simulink model "StPassCmprtMd_MdXX_CrtStat"  (R2018b)
settings: Solver=FixedStepDiscrete  StartTime=0.0  StopTime=10.0  FixedStep=0.01  RelTol=1e-3
settings Model: Creator=sn2xws  LastModifiedBy=sn2xws
settings DataIOCC: SaveFormat=StructureWithTime
settings OptimizationCC: DefaultParameterBehavior=Inlined  EnhancedBackFolding=on  PassReuseOutputArgsAs=Individual arguments  ZeroExternalMemoryAtStartup=off  ZeroInternalMemoryAtStartup=off  OptimizeBlockOrder=speed  DifferentSizesBufferReuse=on  OptimizationCustomize=off
settings DebuggingCC: ParameterTunabilityLossMsg=error
settings ModelReferenceCC: ModelReferenceNumInstancesAllowed=Single
settings SFSimCC: MATLABDynamicMemAlloc=off
settings RTWCC: SystemTargetFile=autosar.tlc  GenCodeOnly=on  TemplateMakefile=ert_default_tmf  Description=AUTOSAR  GenerateReport=on  IncludeHyperlinkInReport=on  LaunchReport=on  GenerateTraceInfo=on  GenerateTraceReport=on  GenerateTraceReportSl=on  GenerateTraceReportSf=on  GenerateTraceReportEml=on
settings CodeAppCC: ForceParamTrailComments=on  IgnoreCustomStorageClasses=off  OperatorAnnotations=on  SimulinkDataObjDesc=on  SFDataObjDesc=on  InsertBlockDesc=on
settings STFCustomTargetCC: TargetLangStandard=C99 (ISO)  MultiwordLength=256  ParMdlRefBuildCompliant=on  CompOptLevelCompliant=on  IncludeMdlTerminateFcn=off  CombineOutputUpdateFcns=on  SuppressErrorStatus=on  ERTCustomFileBanners=on  SupportNonFinite=off  SupportComplex=off  SupportContinuousTime=off  SupportNonInlinedSFcns=off  RemoveResetFunc=on  MATLABClassNameForMDSCustomization=Simulink.SoftwareTarget.ERTCustomization  AutosarCompliant=on  UseToolchainInfoCompliant=on  LookupTableObjectStructAxisOrder=2,1,3,4,...  LUTObjectStructOrderEvenSpacing=Size,Table,Breakpoints  SystemTargetFile=autosar.tlc
settings ERTTargetCC: TargetLangStandard=C99 (ISO)  ConcurrentExecutionCompliant=off  IncludeMdlTerminateFcn=off  SuppressErrorStatus=on  SupportNonFinite=off  SupportComplex=off  ModelStepFunctionPrototypeControlCompliant=off  CPPClassGenCompliant=off  AutosarCompliant=on  LookupTableObjectStructAxisOrder=2,1,3,4,...  LUTObjectStructOrderEvenSpacing=Size,Table,Breakpoints  InlinedParameterPlacement=NonHierarchical  ERTCustomFileTemplate=example_file_process.tlc

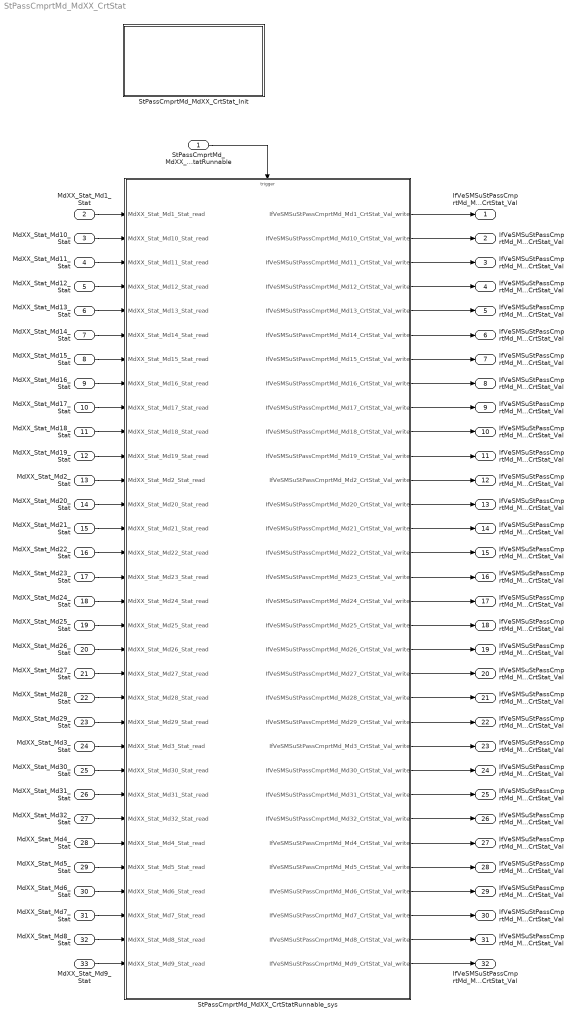
== system StPassCmprtMd_MdXX_CrtStat ==
  StPassCmprtMd_MdXX_CrtStatRunnable : Inport  SampleTime=0.01  OutputFunctionCall=on
  MdXX_Stat_Md1_Stat : Inport  Port=2  OutDataTypeStr=uint8  PortDimensions=1
  MdXX_Stat_Md10_Stat : Inport  Port=3  OutDataTypeStr=uint8  PortDimensions=1
  MdXX_Stat_Md11_Stat : Inport  Port=4  OutDataTypeStr=uint8  PortDimensions=1
  MdXX_Stat_Md12_Stat : Inport  Port=5  OutDataTypeStr=uint8  PortDimensions=1
  MdXX_Stat_Md13_Stat : Inport  Port=6  OutDataTypeStr=uint8  PortDimensions=1
  MdXX_Stat_Md14_Stat : Inport  Port=7  OutDataTypeStr=uint8  PortDimensions=1
  MdXX_Stat_Md15_Stat : Inport  Port=8  OutDataTypeStr=uint8  PortDimensions=1
  MdXX_Stat_Md16_Stat : Inport  Port=9  OutDataTypeStr=uint8  PortDimensions=1
  MdXX_Stat_Md17_Stat : Inport  Port=10  OutDataTypeStr=uint8  PortDimensions=1
  MdXX_Stat_Md18_Stat : Inport  Port=11  OutDataTypeStr=uint8  PortDimensions=1
  MdXX_Stat_Md19_Stat : Inport  Port=12  OutDataTypeStr=uint8  PortDimensions=1
  MdXX_Stat_Md2_Stat : Inport  Port=13  OutDataTypeStr=uint8  PortDimensions=1
  MdXX_Stat_Md20_Stat : Inport  Port=14  OutDataTypeStr=uint8  PortDimensions=1
  MdXX_Stat_Md21_Stat : Inport  Port=15  OutDataTypeStr=uint8  PortDimensions=1
  MdXX_Stat_Md22_Stat : Inport  Port=16  OutDataTypeStr=uint8  PortDimensions=1
  MdXX_Stat_Md23_Stat : Inport  Port=17  OutDataTypeStr=uint8  PortDimensions=1
  MdXX_Stat_Md24_Stat : Inport  Port=18  OutDataTypeStr=uint8  PortDimensions=1
  MdXX_Stat_Md25_Stat : Inport  Port=19  OutDataTypeStr=uint8  PortDimensions=1
  MdXX_Stat_Md26_Stat : Inport  Port=20  OutDataTypeStr=uint8  PortDimensions=1
  MdXX_Stat_Md27_Stat : Inport  Port=21  OutDataTypeStr=uint8  PortDimensions=1
  MdXX_Stat_Md28_Stat : Inport  Port=22  OutDataTypeStr=uint8  PortDimensions=1
  MdXX_Stat_Md29_Stat : Inport  Port=23  OutDataTypeStr=uint8  PortDimensions=1
  MdXX_Stat_Md3_Stat : Inport  Port=24  OutDataTypeStr=uint8  PortDimensions=1
  MdXX_Stat_Md30_Stat : Inport  Port=25  OutDataTypeStr=uint8  PortDimensions=1
  MdXX_Stat_Md31_Stat : Inport  Port=26  OutDataTypeStr=uint8  PortDimensions=1
  MdXX_Stat_Md32_Stat : Inport  Port=27  OutDataTypeStr=uint8  PortDimensions=1
  MdXX_Stat_Md4_Stat : Inport  Port=28  OutDataTypeStr=uint8  PortDimensions=1
  MdXX_Stat_Md5_Stat : Inport  Port=29  OutDataTypeStr=uint8  PortDimensions=1
  MdXX_Stat_Md6_Stat : Inport  Port=30  OutDataTypeStr=uint8  PortDimensions=1
  MdXX_Stat_Md7_Stat : Inport  Port=31  OutDataTypeStr=uint8  PortDimensions=1
  MdXX_Stat_Md8_Stat : Inport  Port=32  OutDataTypeStr=uint8  PortDimensions=1
  MdXX_Stat_Md9_Stat : Inport  Port=33  OutDataTypeStr=uint8  PortDimensions=1
  StPassCmprtMd_MdXX_CrtStatRunnable_sys : Subsystem
  StPassCmprtMd_MdXX_CrtStat_Init : Subsystem
  IfVeSMSuStPassCmprtMd_Md1_CrtStat_Val : Outport  OutDataTypeStr=uint8  PortDimensions=1
  IfVeSMSuStPassCmprtMd_Md10_CrtStat_Val : Outport  Port=2  OutDataTypeStr=uint8  PortDimensions=1
  IfVeSMSuStPassCmprtMd_Md11_CrtStat_Val : Outport  Port=3  OutDataTypeStr=uint8  PortDimensions=1
  IfVeSMSuStPassCmprtMd_Md12_CrtStat_Val : Outport  Port=4  OutDataTypeStr=uint8  PortDimensions=1
  IfVeSMSuStPassCmprtMd_Md13_CrtStat_Val : Outport  Port=5  OutDataTypeStr=uint8  PortDimensions=1
  IfVeSMSuStPassCmprtMd_Md14_CrtStat_Val : Outport  Port=6  OutDataTypeStr=uint8  PortDimensions=1
  IfVeSMSuStPassCmprtMd_Md15_CrtStat_Val : Outport  Port=7  OutDataTypeStr=uint8  PortDimensions=1
  IfVeSMSuStPassCmprtMd_Md16_CrtStat_Val : Outport  Port=8  OutDataTypeStr=uint8  PortDimensions=1
  IfVeSMSuStPassCmprtMd_Md17_CrtStat_Val : Outport  Port=9  OutDataTypeStr=uint8  PortDimensions=1
  IfVeSMSuStPassCmprtMd_Md18_CrtStat_Val : Outport  Port=10  OutDataTypeStr=uint8  PortDimensions=1
  IfVeSMSuStPassCmprtMd_Md19_CrtStat_Val : Outport  Port=11  OutDataTypeStr=uint8  PortDimensions=1
  IfVeSMSuStPassCmprtMd_Md2_CrtStat_Val : Outport  Port=12  OutDataTypeStr=uint8  PortDimensions=1
  IfVeSMSuStPassCmprtMd_Md20_CrtStat_Val : Outport  Port=13  OutDataTypeStr=uint8  PortDimensions=1
  IfVeSMSuStPassCmprtMd_Md21_CrtStat_Val : Outport  Port=14  OutDataTypeStr=uint8  PortDimensions=1
  IfVeSMSuStPassCmprtMd_Md22_CrtStat_Val : Outport  Port=15  OutDataTypeStr=uint8  PortDimensions=1
  IfVeSMSuStPassCmprtMd_Md23_CrtStat_Val : Outport  Port=16  OutDataTypeStr=uint8  PortDimensions=1
  IfVeSMSuStPassCmprtMd_Md24_CrtStat_Val : Outport  Port=17  OutDataTypeStr=uint8  PortDimensions=1
  IfVeSMSuStPassCmprtMd_Md25_CrtStat_Val : Outport  Port=18  OutDataTypeStr=uint8  PortDimensions=1
  IfVeSMSuStPassCmprtMd_Md26_CrtStat_Val : Outport  Port=19  OutDataTypeStr=uint8  PortDimensions=1
  IfVeSMSuStPassCmprtMd_Md27_CrtStat_Val : Outport  Port=20  OutDataTypeStr=uint8  PortDimensions=1
  IfVeSMSuStPassCmprtMd_Md28_CrtStat_Val : Outport  Port=21  OutDataTypeStr=uint8  PortDimensions=1
  IfVeSMSuStPassCmprtMd_Md29_CrtStat_Val : Outport  Port=22  OutDataTypeStr=uint8  PortDimensions=1
  IfVeSMSuStPassCmprtMd_Md3_CrtStat_Val : Outport  Port=23  OutDataTypeStr=uint8  PortDimensions=1
  IfVeSMSuStPassCmprtMd_Md30_CrtStat_Val : Outport  Port=24  OutDataTypeStr=uint8  PortDimensions=1
  IfVeSMSuStPassCmprtMd_Md31_CrtStat_Val : Outport  Port=25  OutDataTypeStr=uint8  PortDimensions=1
  IfVeSMSuStPassCmprtMd_Md32_CrtStat_Val : Outport  Port=26  OutDataTypeStr=uint8  PortDimensions=1
  IfVeSMSuStPassCmprtMd_Md4_CrtStat_Val : Outport  Port=27  OutDataTypeStr=uint8  PortDimensions=1
  IfVeSMSuStPassCmprtMd_Md5_CrtStat_Val : Outport  Port=28  OutDataTypeStr=uint8  PortDimensions=1
  IfVeSMSuStPassCmprtMd_Md6_CrtStat_Val : Outport  Port=29  OutDataTypeStr=uint8  PortDimensions=1
  IfVeSMSuStPassCmprtMd_Md7_CrtStat_Val : Outport  Port=30  OutDataTypeStr=uint8  PortDimensions=1
  IfVeSMSuStPassCmprtMd_Md8_CrtStat_Val : Outport  Port=31  OutDataTypeStr=uint8  PortDimensions=1
  IfVeSMSuStPassCmprtMd_Md9_CrtStat_Val : Outport  Port=32  OutDataTypeStr=uint8  PortDimensions=1
  wires:
  MdXX_Stat_Md1_Stat/1 -> StPassCmprtMd_MdXX_CrtStatRunnable_sys/1(MdXX_Stat_Md1_Stat_read)
  MdXX_Stat_Md10_Stat/1 -> StPassCmprtMd_MdXX_CrtStatRunnable_sys/2(MdXX_Stat_Md10_Stat_read)
  MdXX_Stat_Md11_Stat/1 -> StPassCmprtMd_MdXX_CrtStatRunnable_sys/3(MdXX_Stat_Md11_Stat_read)
  MdXX_Stat_Md12_Stat/1 -> StPassCmprtMd_MdXX_CrtStatRunnable_sys/4(MdXX_Stat_Md12_Stat_read)
  MdXX_Stat_Md13_Stat/1 -> StPassCmprtMd_MdXX_CrtStatRunnable_sys/5(MdXX_Stat_Md13_Stat_read)
  MdXX_Stat_Md14_Stat/1 -> StPassCmprtMd_MdXX_CrtStatRunnable_sys/6(MdXX_Stat_Md14_Stat_read)
  MdXX_Stat_Md15_Stat/1 -> StPassCmprtMd_MdXX_CrtStatRunnable_sys/7(MdXX_Stat_Md15_Stat_read)
  MdXX_Stat_Md16_Stat/1 -> StPassCmprtMd_MdXX_CrtStatRunnable_sys/8(MdXX_Stat_Md16_Stat_read)
  MdXX_Stat_Md17_Stat/1 -> StPassCmprtMd_MdXX_CrtStatRunnable_sys/9(MdXX_Stat_Md17_Stat_read)
  MdXX_Stat_Md18_Stat/1 -> StPassCmprtMd_MdXX_CrtStatRunnable_sys/10(MdXX_Stat_Md18_Stat_read)
  MdXX_Stat_Md19_Stat/1 -> StPassCmprtMd_MdXX_CrtStatRunnable_sys/11(MdXX_Stat_Md19_Stat_read)
  MdXX_Stat_Md2_Stat/1 -> StPassCmprtMd_MdXX_CrtStatRunnable_sys/12(MdXX_Stat_Md2_Stat_read)
  MdXX_Stat_Md20_Stat/1 -> StPassCmprtMd_MdXX_CrtStatRunnable_sys/13(MdXX_Stat_Md20_Stat_read)
  MdXX_Stat_Md21_Stat/1 -> StPassCmprtMd_MdXX_CrtStatRunnable_sys/14(MdXX_Stat_Md21_Stat_read)
  MdXX_Stat_Md22_Stat/1 -> StPassCmprtMd_MdXX_CrtStatRunnable_sys/15(MdXX_Stat_Md22_Stat_read)
  MdXX_Stat_Md23_Stat/1 -> StPassCmprtMd_MdXX_CrtStatRunnable_sys/16(MdXX_Stat_Md23_Stat_read)
  MdXX_Stat_Md24_Stat/1 -> StPassCmprtMd_MdXX_CrtStatRunnable_sys/17(MdXX_Stat_Md24_Stat_read)
  MdXX_Stat_Md25_Stat/1 -> StPassCmprtMd_MdXX_CrtStatRunnable_sys/18(MdXX_Stat_Md25_Stat_read)
  MdXX_Stat_Md26_Stat/1 -> StPassCmprtMd_MdXX_CrtStatRunnable_sys/19(MdXX_Stat_Md26_Stat_read)
  MdXX_Stat_Md27_Stat/1 -> StPassCmprtMd_MdXX_CrtStatRunnable_sys/20(MdXX_Stat_Md27_Stat_read)
  MdXX_Stat_Md28_Stat/1 -> StPassCmprtMd_MdXX_CrtStatRunnable_sys/21(MdXX_Stat_Md28_Stat_read)
  MdXX_Stat_Md29_Stat/1 -> StPassCmprtMd_MdXX_CrtStatRunnable_sys/22(MdXX_Stat_Md29_Stat_read)
  MdXX_Stat_Md3_Stat/1 -> StPassCmprtMd_MdXX_CrtStatRunnable_sys/23(MdXX_Stat_Md3_Stat_read)
  MdXX_Stat_Md30_Stat/1 -> StPassCmprtMd_MdXX_CrtStatRunnable_sys/24(MdXX_Stat_Md30_Stat_read)
  MdXX_Stat_Md31_Stat/1 -> StPassCmprtMd_MdXX_CrtStatRunnable_sys/25(MdXX_Stat_Md31_Stat_read)
  MdXX_Stat_Md32_Stat/1 -> StPassCmprtMd_MdXX_CrtStatRunnable_sys/26(MdXX_Stat_Md32_Stat_read)
  MdXX_Stat_Md4_Stat/1 -> StPassCmprtMd_MdXX_CrtStatRunnable_sys/27(MdXX_Stat_Md4_Stat_read)
  MdXX_Stat_Md5_Stat/1 -> StPassCmprtMd_MdXX_CrtStatRunnable_sys/28(MdXX_Stat_Md5_Stat_read)
  MdXX_Stat_Md6_Stat/1 -> StPassCmprtMd_MdXX_CrtStatRunnable_sys/29(MdXX_Stat_Md6_Stat_read)
  MdXX_Stat_Md7_Stat/1 -> StPassCmprtMd_MdXX_CrtStatRunnable_sys/30(MdXX_Stat_Md7_Stat_read)
  MdXX_Stat_Md8_Stat/1 -> StPassCmprtMd_MdXX_CrtStatRunnable_sys/31(MdXX_Stat_Md8_Stat_read)
  MdXX_Stat_Md9_Stat/1 -> StPassCmprtMd_MdXX_CrtStatRunnable_sys/32(MdXX_Stat_Md9_Stat_read)
  StPassCmprtMd_MdXX_CrtStatRunnable_sys/1(IfVeSMSuStPassCmprtMd_Md1_CrtStat_Val_write) -> IfVeSMSuStPassCmprtMd_Md1_CrtStat_Val/1
  StPassCmprtMd_MdXX_CrtStatRunnable_sys/2(IfVeSMSuStPassCmprtMd_Md10_CrtStat_Val_write) -> IfVeSMSuStPassCmprtMd_Md10_CrtStat_Val/1
  StPassCmprtMd_MdXX_CrtStatRunnable_sys/3(IfVeSMSuStPassCmprtMd_Md11_CrtStat_Val_write) -> IfVeSMSuStPassCmprtMd_Md11_CrtStat_Val/1
  StPassCmprtMd_MdXX_CrtStatRunnable_sys/4(IfVeSMSuStPassCmprtMd_Md12_CrtStat_Val_write) -> IfVeSMSuStPassCmprtMd_Md12_CrtStat_Val/1
  StPassCmprtMd_MdXX_CrtStatRunnable_sys/5(IfVeSMSuStPassCmprtMd_Md13_CrtStat_Val_write) -> IfVeSMSuStPassCmprtMd_Md13_CrtStat_Val/1
  StPassCmprtMd_MdXX_CrtStatRunnable_sys/6(IfVeSMSuStPassCmprtMd_Md14_CrtStat_Val_write) -> IfVeSMSuStPassCmprtMd_Md14_CrtStat_Val/1
  StPassCmprtMd_MdXX_CrtStatRunnable_sys/7(IfVeSMSuStPassCmprtMd_Md15_CrtStat_Val_write) -> IfVeSMSuStPassCmprtMd_Md15_CrtStat_Val/1
  StPassCmprtMd_MdXX_CrtStatRunnable_sys/8(IfVeSMSuStPassCmprtMd_Md16_CrtStat_Val_write) -> IfVeSMSuStPassCmprtMd_Md16_CrtStat_Val/1
  StPassCmprtMd_MdXX_CrtStatRunnable_sys/9(IfVeSMSuStPassCmprtMd_Md17_CrtStat_Val_write) -> IfVeSMSuStPassCmprtMd_Md17_CrtStat_Val/1
  StPassCmprtMd_MdXX_CrtStatRunnable_sys/10(IfVeSMSuStPassCmprtMd_Md18_CrtStat_Val_write) -> IfVeSMSuStPassCmprtMd_Md18_CrtStat_Val/1
  StPassCmprtMd_MdXX_CrtStatRunnable_sys/11(IfVeSMSuStPassCmprtMd_Md19_CrtStat_Val_write) -> IfVeSMSuStPassCmprtMd_Md19_CrtStat_Val/1
  StPassCmprtMd_MdXX_CrtStatRunnable_sys/12(IfVeSMSuStPassCmprtMd_Md2_CrtStat_Val_write) -> IfVeSMSuStPassCmprtMd_Md2_CrtStat_Val/1
  StPassCmprtMd_MdXX_CrtStatRunnable_sys/13(IfVeSMSuStPassCmprtMd_Md20_CrtStat_Val_write) -> IfVeSMSuStPassCmprtMd_Md20_CrtStat_Val/1
  StPassCmprtMd_MdXX_CrtStatRunnable_sys/14(IfVeSMSuStPassCmprtMd_Md21_CrtStat_Val_write) -> IfVeSMSuStPassCmprtMd_Md21_CrtStat_Val/1
  StPassCmprtMd_MdXX_CrtStatRunnable_sys/15(IfVeSMSuStPassCmprtMd_Md22_CrtStat_Val_write) -> IfVeSMSuStPassCmprtMd_Md22_CrtStat_Val/1
  StPassCmprtMd_MdXX_CrtStatRunnable_sys/16(IfVeSMSuStPassCmprtMd_Md23_CrtStat_Val_write) -> IfVeSMSuStPassCmprtMd_Md23_CrtStat_Val/1
  StPassCmprtMd_MdXX_CrtStatRunnable_sys/17(IfVeSMSuStPassCmprtMd_Md24_CrtStat_Val_write) -> IfVeSMSuStPassCmprtMd_Md24_CrtStat_Val/1
  StPassCmprtMd_MdXX_CrtStatRunnable_sys/18(IfVeSMSuStPassCmprtMd_Md25_CrtStat_Val_write) -> IfVeSMSuStPassCmprtMd_Md25_CrtStat_Val/1
  StPassCmprtMd_MdXX_CrtStatRunnable_sys/19(IfVeSMSuStPassCmprtMd_Md26_CrtStat_Val_write) -> IfVeSMSuStPassCmprtMd_Md26_CrtStat_Val/1
  StPassCmprtMd_MdXX_CrtStatRunnable_sys/20(IfVeSMSuStPassCmprtMd_Md27_CrtStat_Val_write) -> IfVeSMSuStPassCmprtMd_Md27_CrtStat_Val/1
  StPassCmprtMd_MdXX_CrtStatRunnable_sys/21(IfVeSMSuStPassCmprtMd_Md28_CrtStat_Val_write) -> IfVeSMSuStPassCmprtMd_Md28_CrtStat_Val/1
  StPassCmprtMd_MdXX_CrtStatRunnable_sys/22(IfVeSMSuStPassCmprtMd_Md29_CrtStat_Val_write) -> IfVeSMSuStPassCmprtMd_Md29_CrtStat_Val/1
  StPassCmprtMd_MdXX_CrtStatRunnable_sys/23(IfVeSMSuStPassCmprtMd_Md3_CrtStat_Val_write) -> IfVeSMSuStPassCmprtMd_Md3_CrtStat_Val/1
  StPassCmprtMd_MdXX_CrtStatRunnable_sys/24(IfVeSMSuStPassCmprtMd_Md30_CrtStat_Val_write) -> IfVeSMSuStPassCmprtMd_Md30_CrtStat_Val/1
  StPassCmprtMd_MdXX_CrtStatRunnable_sys/25(IfVeSMSuStPassCmprtMd_Md31_CrtStat_Val_write) -> IfVeSMSuStPassCmprtMd_Md31_CrtStat_Val/1
  StPassCmprtMd_MdXX_CrtStatRunnable_sys/26(IfVeSMSuStPassCmprtMd_Md32_CrtStat_Val_write) -> IfVeSMSuStPassCmprtMd_Md32_CrtStat_Val/1
  StPassCmprtMd_MdXX_CrtStatRunnable_sys/27(IfVeSMSuStPassCmprtMd_Md4_CrtStat_Val_write) -> IfVeSMSuStPassCmprtMd_Md4_CrtStat_Val/1
  StPassCmprtMd_MdXX_CrtStatRunnable_sys/28(IfVeSMSuStPassCmprtMd_Md5_CrtStat_Val_write) -> IfVeSMSuStPassCmprtMd_Md5_CrtStat_Val/1
  StPassCmprtMd_MdXX_CrtStatRunnable_sys/29(IfVeSMSuStPassCmprtMd_Md6_CrtStat_Val_write) -> IfVeSMSuStPassCmprtMd_Md6_CrtStat_Val/1
  StPassCmprtMd_MdXX_CrtStatRunnable_sys/30(IfVeSMSuStPassCmprtMd_Md7_CrtStat_Val_write) -> IfVeSMSuStPassCmprtMd_Md7_CrtStat_Val/1
  StPassCmprtMd_MdXX_CrtStatRunnable_sys/31(IfVeSMSuStPassCmprtMd_Md8_CrtStat_Val_write) -> IfVeSMSuStPassCmprtMd_Md8_CrtStat_Val/1
  StPassCmprtMd_MdXX_CrtStatRunnable_sys/32(IfVeSMSuStPassCmprtMd_Md9_CrtStat_Val_write) -> IfVeSMSuStPassCmprtMd_Md9_CrtStat_Val/1
  StPassCmprtMd_MdXX_CrtStatRunnable/1 -> StPassCmprtMd_MdXX_CrtStatRunnable_sys/Trigger

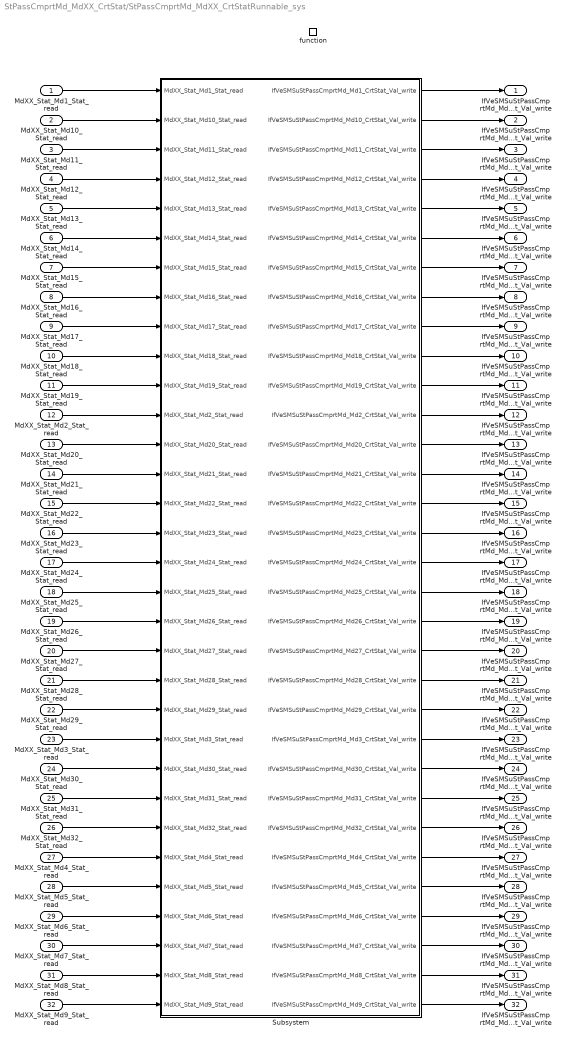
== system StPassCmprtMd_MdXX_CrtStat/StPassCmprtMd_MdXX_CrtStatRunnable_sys ==
  MdXX_Stat_Md1_Stat_read : Inport
  MdXX_Stat_Md10_Stat_read : Inport  Port=2
  MdXX_Stat_Md11_Stat_read : Inport  Port=3
  MdXX_Stat_Md12_Stat_read : Inport  Port=4
  MdXX_Stat_Md13_Stat_read : Inport  Port=5
  MdXX_Stat_Md14_Stat_read : Inport  Port=6
  MdXX_Stat_Md15_Stat_read : Inport  Port=7
  MdXX_Stat_Md16_Stat_read : Inport  Port=8
  MdXX_Stat_Md17_Stat_read : Inport  Port=9
  MdXX_Stat_Md18_Stat_read : Inport  Port=10
  MdXX_Stat_Md19_Stat_read : Inport  Port=11
  MdXX_Stat_Md2_Stat_read : Inport  Port=12
  MdXX_Stat_Md20_Stat_read : Inport  Port=13
  MdXX_Stat_Md21_Stat_read : Inport  Port=14
  MdXX_Stat_Md22_Stat_read : Inport  Port=15
  MdXX_Stat_Md23_Stat_read : Inport  Port=16
  MdXX_Stat_Md24_Stat_read : Inport  Port=17
  MdXX_Stat_Md25_Stat_read : Inport  Port=18
  MdXX_Stat_Md26_Stat_read : Inport  Port=19
  MdXX_Stat_Md27_Stat_read : Inport  Port=20
  MdXX_Stat_Md28_Stat_read : Inport  Port=21
  MdXX_Stat_Md29_Stat_read : Inport  Port=22
  MdXX_Stat_Md3_Stat_read : Inport  Port=23
  MdXX_Stat_Md30_Stat_read : Inport  Port=24
  MdXX_Stat_Md31_Stat_read : Inport  Port=25
  MdXX_Stat_Md32_Stat_read : Inport  Port=26
  MdXX_Stat_Md4_Stat_read : Inport  Port=27
  MdXX_Stat_Md5_Stat_read : Inport  Port=28
  MdXX_Stat_Md6_Stat_read : Inport  Port=29
  MdXX_Stat_Md7_Stat_read : Inport  Port=30
  MdXX_Stat_Md8_Stat_read : Inport  Port=31
  MdXX_Stat_Md9_Stat_read : Inport  Port=32
  function : TriggerPort  TriggerType=function-call  VariantControl=(inherit)  SampleTimeType=periodic  SampleTime=-1
  Subsystem : Subsystem
  IfVeSMSuStPassCmprtMd_Md1_CrtStat_Val_write : Outport
      settings: EnsureOutportIsVirtual=on
  IfVeSMSuStPassCmprtMd_Md10_CrtStat_Val_write : Outport  Port=2
      settings: EnsureOutportIsVirtual=on
  IfVeSMSuStPassCmprtMd_Md11_CrtStat_Val_write : Outport  Port=3
      settings: EnsureOutportIsVirtual=on
  IfVeSMSuStPassCmprtMd_Md12_CrtStat_Val_write : Outport  Port=4
      settings: EnsureOutportIsVirtual=on
  IfVeSMSuStPassCmprtMd_Md13_CrtStat_Val_write : Outport  Port=5
      settings: EnsureOutportIsVirtual=on
  IfVeSMSuStPassCmprtMd_Md14_CrtStat_Val_write : Outport  Port=6
      settings: EnsureOutportIsVirtual=on
  IfVeSMSuStPassCmprtMd_Md15_CrtStat_Val_write : Outport  Port=7
      settings: EnsureOutportIsVirtual=on
  IfVeSMSuStPassCmprtMd_Md16_CrtStat_Val_write : Outport  Port=8
      settings: EnsureOutportIsVirtual=on
  IfVeSMSuStPassCmprtMd_Md17_CrtStat_Val_write : Outport  Port=9
      settings: EnsureOutportIsVirtual=on
  IfVeSMSuStPassCmprtMd_Md18_CrtStat_Val_write : Outport  Port=10
      settings: EnsureOutportIsVirtual=on
  IfVeSMSuStPassCmprtMd_Md19_CrtStat_Val_write : Outport  Port=11
      settings: EnsureOutportIsVirtual=on
  IfVeSMSuStPassCmprtMd_Md2_CrtStat_Val_write : Outport  Port=12
      settings: EnsureOutportIsVirtual=on
  IfVeSMSuStPassCmprtMd_Md20_CrtStat_Val_write : Outport  Port=13
      settings: EnsureOutportIsVirtual=on
  IfVeSMSuStPassCmprtMd_Md21_CrtStat_Val_write : Outport  Port=14
      settings: EnsureOutportIsVirtual=on
  IfVeSMSuStPassCmprtMd_Md22_CrtStat_Val_write : Outport  Port=15
      settings: EnsureOutportIsVirtual=on
  IfVeSMSuStPassCmprtMd_Md23_CrtStat_Val_write : Outport  Port=16
      settings: EnsureOutportIsVirtual=on
  IfVeSMSuStPassCmprtMd_Md24_CrtStat_Val_write : Outport  Port=17
      settings: EnsureOutportIsVirtual=on
  IfVeSMSuStPassCmprtMd_Md25_CrtStat_Val_write : Outport  Port=18
      settings: EnsureOutportIsVirtual=on
  IfVeSMSuStPassCmprtMd_Md26_CrtStat_Val_write : Outport  Port=19
      settings: EnsureOutportIsVirtual=on
  IfVeSMSuStPassCmprtMd_Md27_CrtStat_Val_write : Outport  Port=20
      settings: EnsureOutportIsVirtual=on
  IfVeSMSuStPassCmprtMd_Md28_CrtStat_Val_write : Outport  Port=21
      settings: EnsureOutportIsVirtual=on
  IfVeSMSuStPassCmprtMd_Md29_CrtStat_Val_write : Outport  Port=22
      settings: EnsureOutportIsVirtual=on
  IfVeSMSuStPassCmprtMd_Md3_CrtStat_Val_write : Outport  Port=23
      settings: EnsureOutportIsVirtual=on
  IfVeSMSuStPassCmprtMd_Md30_CrtStat_Val_write : Outport  Port=24
      settings: EnsureOutportIsVirtual=on
  IfVeSMSuStPassCmprtMd_Md31_CrtStat_Val_write : Outport  Port=25
      settings: EnsureOutportIsVirtual=on
  IfVeSMSuStPassCmprtMd_Md32_CrtStat_Val_write : Outport  Port=26
      settings: EnsureOutportIsVirtual=on
  IfVeSMSuStPassCmprtMd_Md4_CrtStat_Val_write : Outport  Port=27
      settings: EnsureOutportIsVirtual=on
  IfVeSMSuStPassCmprtMd_Md5_CrtStat_Val_write : Outport  Port=28
      settings: EnsureOutportIsVirtual=on
  IfVeSMSuStPassCmprtMd_Md6_CrtStat_Val_write : Outport  Port=29
      settings: EnsureOutportIsVirtual=on
  IfVeSMSuStPassCmprtMd_Md7_CrtStat_Val_write : Outport  Port=30
      settings: EnsureOutportIsVirtual=on
  IfVeSMSuStPassCmprtMd_Md8_CrtStat_Val_write : Outport  Port=31
      settings: EnsureOutportIsVirtual=on
  IfVeSMSuStPassCmprtMd_Md9_CrtStat_Val_write : Outport  Port=32
      settings: EnsureOutportIsVirtual=on
  wires:
  MdXX_Stat_Md1_Stat_read/1 -> Subsystem/1(MdXX_Stat_Md1_Stat_read)
  MdXX_Stat_Md10_Stat_read/1 -> Subsystem/2(MdXX_Stat_Md10_Stat_read)
  MdXX_Stat_Md11_Stat_read/1 -> Subsystem/3(MdXX_Stat_Md11_Stat_read)
  MdXX_Stat_Md12_Stat_read/1 -> Subsystem/4(MdXX_Stat_Md12_Stat_read)
  MdXX_Stat_Md13_Stat_read/1 -> Subsystem/5(MdXX_Stat_Md13_Stat_read)
  MdXX_Stat_Md14_Stat_read/1 -> Subsystem/6(MdXX_Stat_Md14_Stat_read)
  MdXX_Stat_Md15_Stat_read/1 -> Subsystem/7(MdXX_Stat_Md15_Stat_read)
  MdXX_Stat_Md16_Stat_read/1 -> Subsystem/8(MdXX_Stat_Md16_Stat_read)
  MdXX_Stat_Md17_Stat_read/1 -> Subsystem/9(MdXX_Stat_Md17_Stat_read)
  MdXX_Stat_Md18_Stat_read/1 -> Subsystem/10(MdXX_Stat_Md18_Stat_read)
  MdXX_Stat_Md19_Stat_read/1 -> Subsystem/11(MdXX_Stat_Md19_Stat_read)
  MdXX_Stat_Md2_Stat_read/1 -> Subsystem/12(MdXX_Stat_Md2_Stat_read)
  MdXX_Stat_Md20_Stat_read/1 -> Subsystem/13(MdXX_Stat_Md20_Stat_read)
  MdXX_Stat_Md21_Stat_read/1 -> Subsystem/14(MdXX_Stat_Md21_Stat_read)
  MdXX_Stat_Md22_Stat_read/1 -> Subsystem/15(MdXX_Stat_Md22_Stat_read)
  MdXX_Stat_Md23_Stat_read/1 -> Subsystem/16(MdXX_Stat_Md23_Stat_read)
  MdXX_Stat_Md24_Stat_read/1 -> Subsystem/17(MdXX_Stat_Md24_Stat_read)
  MdXX_Stat_Md25_Stat_read/1 -> Subsystem/18(MdXX_Stat_Md25_Stat_read)
  MdXX_Stat_Md26_Stat_read/1 -> Subsystem/19(MdXX_Stat_Md26_Stat_read)
  MdXX_Stat_Md27_Stat_read/1 -> Subsystem/20(MdXX_Stat_Md27_Stat_read)
  MdXX_Stat_Md28_Stat_read/1 -> Subsystem/21(MdXX_Stat_Md28_Stat_read)
  MdXX_Stat_Md29_Stat_read/1 -> Subsystem/22(MdXX_Stat_Md29_Stat_read)
  MdXX_Stat_Md3_Stat_read/1 -> Subsystem/23(MdXX_Stat_Md3_Stat_read)
  MdXX_Stat_Md30_Stat_read/1 -> Subsystem/24(MdXX_Stat_Md30_Stat_read)
  MdXX_Stat_Md31_Stat_read/1 -> Subsystem/25(MdXX_Stat_Md31_Stat_read)
  MdXX_Stat_Md32_Stat_read/1 -> Subsystem/26(MdXX_Stat_Md32_Stat_read)
  MdXX_Stat_Md4_Stat_read/1 -> Subsystem/27(MdXX_Stat_Md4_Stat_read)
  MdXX_Stat_Md5_Stat_read/1 -> Subsystem/28(MdXX_Stat_Md5_Stat_read)
  MdXX_Stat_Md6_Stat_read/1 -> Subsystem/29(MdXX_Stat_Md6_Stat_read)
  MdXX_Stat_Md7_Stat_read/1 -> Subsystem/30(MdXX_Stat_Md7_Stat_read)
  MdXX_Stat_Md8_Stat_read/1 -> Subsystem/31(MdXX_Stat_Md8_Stat_read)
  MdXX_Stat_Md9_Stat_read/1 -> Subsystem/32(MdXX_Stat_Md9_Stat_read)
  Subsystem/1(IfVeSMSuStPassCmprtMd_Md1_CrtStat_Val_write) -> IfVeSMSuStPassCmprtMd_Md1_CrtStat_Val_write/1
  Subsystem/2(IfVeSMSuStPassCmprtMd_Md10_CrtStat_Val_write) -> IfVeSMSuStPassCmprtMd_Md10_CrtStat_Val_write/1
  Subsystem/3(IfVeSMSuStPassCmprtMd_Md11_CrtStat_Val_write) -> IfVeSMSuStPassCmprtMd_Md11_CrtStat_Val_write/1
  Subsystem/4(IfVeSMSuStPassCmprtMd_Md12_CrtStat_Val_write) -> IfVeSMSuStPassCmprtMd_Md12_CrtStat_Val_write/1
  Subsystem/5(IfVeSMSuStPassCmprtMd_Md13_CrtStat_Val_write) -> IfVeSMSuStPassCmprtMd_Md13_CrtStat_Val_write/1
  Subsystem/6(IfVeSMSuStPassCmprtMd_Md14_CrtStat_Val_write) -> IfVeSMSuStPassCmprtMd_Md14_CrtStat_Val_write/1
  Subsystem/7(IfVeSMSuStPassCmprtMd_Md15_CrtStat_Val_write) -> IfVeSMSuStPassCmprtMd_Md15_CrtStat_Val_write/1
  Subsystem/8(IfVeSMSuStPassCmprtMd_Md16_CrtStat_Val_write) -> IfVeSMSuStPassCmprtMd_Md16_CrtStat_Val_write/1
  Subsystem/9(IfVeSMSuStPassCmprtMd_Md17_CrtStat_Val_write) -> IfVeSMSuStPassCmprtMd_Md17_CrtStat_Val_write/1
  Subsystem/10(IfVeSMSuStPassCmprtMd_Md18_CrtStat_Val_write) -> IfVeSMSuStPassCmprtMd_Md18_CrtStat_Val_write/1
  Subsystem/11(IfVeSMSuStPassCmprtMd_Md19_CrtStat_Val_write) -> IfVeSMSuStPassCmprtMd_Md19_CrtStat_Val_write/1
  Subsystem/12(IfVeSMSuStPassCmprtMd_Md2_CrtStat_Val_write) -> IfVeSMSuStPassCmprtMd_Md2_CrtStat_Val_write/1
  Subsystem/13(IfVeSMSuStPassCmprtMd_Md20_CrtStat_Val_write) -> IfVeSMSuStPassCmprtMd_Md20_CrtStat_Val_write/1
  Subsystem/14(IfVeSMSuStPassCmprtMd_Md21_CrtStat_Val_write) -> IfVeSMSuStPassCmprtMd_Md21_CrtStat_Val_write/1
  Subsystem/15(IfVeSMSuStPassCmprtMd_Md22_CrtStat_Val_write) -> IfVeSMSuStPassCmprtMd_Md22_CrtStat_Val_write/1
  Subsystem/16(IfVeSMSuStPassCmprtMd_Md23_CrtStat_Val_write) -> IfVeSMSuStPassCmprtMd_Md23_CrtStat_Val_write/1
  Subsystem/17(IfVeSMSuStPassCmprtMd_Md24_CrtStat_Val_write) -> IfVeSMSuStPassCmprtMd_Md24_CrtStat_Val_write/1
  Subsystem/18(IfVeSMSuStPassCmprtMd_Md25_CrtStat_Val_write) -> IfVeSMSuStPassCmprtMd_Md25_CrtStat_Val_write/1
  Subsystem/19(IfVeSMSuStPassCmprtMd_Md26_CrtStat_Val_write) -> IfVeSMSuStPassCmprtMd_Md26_CrtStat_Val_write/1
  Subsystem/20(IfVeSMSuStPassCmprtMd_Md27_CrtStat_Val_write) -> IfVeSMSuStPassCmprtMd_Md27_CrtStat_Val_write/1
  Subsystem/21(IfVeSMSuStPassCmprtMd_Md28_CrtStat_Val_write) -> IfVeSMSuStPassCmprtMd_Md28_CrtStat_Val_write/1
  Subsystem/22(IfVeSMSuStPassCmprtMd_Md29_CrtStat_Val_write) -> IfVeSMSuStPassCmprtMd_Md29_CrtStat_Val_write/1
  Subsystem/23(IfVeSMSuStPassCmprtMd_Md3_CrtStat_Val_write) -> IfVeSMSuStPassCmprtMd_Md3_CrtStat_Val_write/1
  Subsystem/24(IfVeSMSuStPassCmprtMd_Md30_CrtStat_Val_write) -> IfVeSMSuStPassCmprtMd_Md30_CrtStat_Val_write/1
  Subsystem/25(IfVeSMSuStPassCmprtMd_Md31_CrtStat_Val_write) -> IfVeSMSuStPassCmprtMd_Md31_CrtStat_Val_write/1
  Subsystem/26(IfVeSMSuStPassCmprtMd_Md32_CrtStat_Val_write) -> IfVeSMSuStPassCmprtMd_Md32_CrtStat_Val_write/1
  Subsystem/27(IfVeSMSuStPassCmprtMd_Md4_CrtStat_Val_write) -> IfVeSMSuStPassCmprtMd_Md4_CrtStat_Val_write/1
  Subsystem/28(IfVeSMSuStPassCmprtMd_Md5_CrtStat_Val_write) -> IfVeSMSuStPassCmprtMd_Md5_CrtStat_Val_write/1
  Subsystem/29(IfVeSMSuStPassCmprtMd_Md6_CrtStat_Val_write) -> IfVeSMSuStPassCmprtMd_Md6_CrtStat_Val_write/1
  Subsystem/30(IfVeSMSuStPassCmprtMd_Md7_CrtStat_Val_write) -> IfVeSMSuStPassCmprtMd_Md7_CrtStat_Val_write/1
  Subsystem/31(IfVeSMSuStPassCmprtMd_Md8_CrtStat_Val_write) -> IfVeSMSuStPassCmprtMd_Md8_CrtStat_Val_write/1
  Subsystem/32(IfVeSMSuStPassCmprtMd_Md9_CrtStat_Val_write) -> IfVeSMSuStPassCmprtMd_Md9_CrtStat_Val_write/1

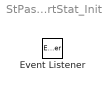
== system StPassCmprtMd_MdXX_CrtStat/StPassCmprtMd_MdXX_CrtStat_Init ==
  Event Listener : EventListener  EventName=reset

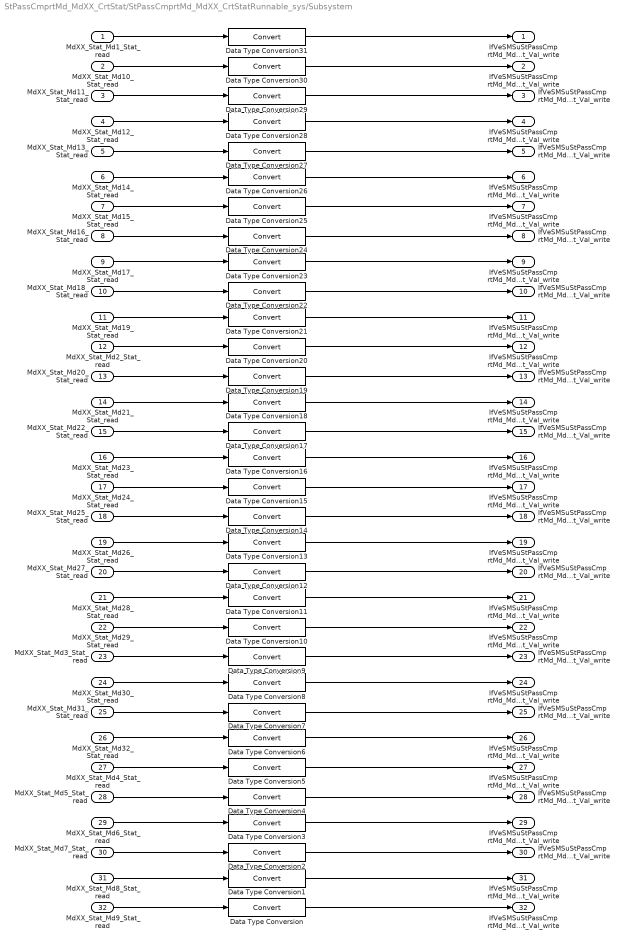
== system StPassCmprtMd_MdXX_CrtStat/StPassCmprtMd_MdXX_CrtStatRunnable_sys/Subsystem ==
  MdXX_Stat_Md1_Stat_read : Inport
  MdXX_Stat_Md10_Stat_read : Inport  Port=2
  MdXX_Stat_Md11_Stat_read : Inport  Port=3
  MdXX_Stat_Md12_Stat_read : Inport  Port=4
  MdXX_Stat_Md13_Stat_read : Inport  Port=5
  MdXX_Stat_Md14_Stat_read : Inport  Port=6
  MdXX_Stat_Md15_Stat_read : Inport  Port=7
  MdXX_Stat_Md16_Stat_read : Inport  Port=8
  MdXX_Stat_Md17_Stat_read : Inport  Port=9
  MdXX_Stat_Md18_Stat_read : Inport  Port=10
  MdXX_Stat_Md19_Stat_read : Inport  Port=11
  MdXX_Stat_Md2_Stat_read : Inport  Port=12
  MdXX_Stat_Md20_Stat_read : Inport  Port=13
  MdXX_Stat_Md21_Stat_read : Inport  Port=14
  MdXX_Stat_Md22_Stat_read : Inport  Port=15
  MdXX_Stat_Md23_Stat_read : Inport  Port=16
  MdXX_Stat_Md24_Stat_read : Inport  Port=17
  MdXX_Stat_Md25_Stat_read : Inport  Port=18
  MdXX_Stat_Md26_Stat_read : Inport  Port=19
  MdXX_Stat_Md27_Stat_read : Inport  Port=20
  MdXX_Stat_Md28_Stat_read : Inport  Port=21
  MdXX_Stat_Md29_Stat_read : Inport  Port=22
  MdXX_Stat_Md3_Stat_read : Inport  Port=23
  MdXX_Stat_Md30_Stat_read : Inport  Port=24
  MdXX_Stat_Md31_Stat_read : Inport  Port=25
  MdXX_Stat_Md32_Stat_read : Inport  Port=26
  MdXX_Stat_Md4_Stat_read : Inport  Port=27
  MdXX_Stat_Md5_Stat_read : Inport  Port=28
  MdXX_Stat_Md6_Stat_read : Inport  Port=29
  MdXX_Stat_Md7_Stat_read : Inport  Port=30
  MdXX_Stat_Md8_Stat_read : Inport  Port=31
  MdXX_Stat_Md9_Stat_read : Inport  Port=32
  Data Type Conversion{,1..31} (32 alike) : DataTypeConversion
  IfVeSMSuStPassCmprtMd_Md1_CrtStat_Val_write : Outport
      settings: EnsureOutportIsVirtual=on
  IfVeSMSuStPassCmprtMd_Md10_CrtStat_Val_write : Outport  Port=2
      settings: EnsureOutportIsVirtual=on
  IfVeSMSuStPassCmprtMd_Md11_CrtStat_Val_write : Outport  Port=3
      settings: EnsureOutportIsVirtual=on
  IfVeSMSuStPassCmprtMd_Md12_CrtStat_Val_write : Outport  Port=4
      settings: EnsureOutportIsVirtual=on
  IfVeSMSuStPassCmprtMd_Md13_CrtStat_Val_write : Outport  Port=5
      settings: EnsureOutportIsVirtual=on
  IfVeSMSuStPassCmprtMd_Md14_CrtStat_Val_write : Outport  Port=6
      settings: EnsureOutportIsVirtual=on
  IfVeSMSuStPassCmprtMd_Md15_CrtStat_Val_write : Outport  Port=7
      settings: EnsureOutportIsVirtual=on
  IfVeSMSuStPassCmprtMd_Md16_CrtStat_Val_write : Outport  Port=8
      settings: EnsureOutportIsVirtual=on
  IfVeSMSuStPassCmprtMd_Md17_CrtStat_Val_write : Outport  Port=9
      settings: EnsureOutportIsVirtual=on
  IfVeSMSuStPassCmprtMd_Md18_CrtStat_Val_write : Outport  Port=10
      settings: EnsureOutportIsVirtual=on
  IfVeSMSuStPassCmprtMd_Md19_CrtStat_Val_write : Outport  Port=11
      settings: EnsureOutportIsVirtual=on
  IfVeSMSuStPassCmprtMd_Md2_CrtStat_Val_write : Outport  Port=12
      settings: EnsureOutportIsVirtual=on
  IfVeSMSuStPassCmprtMd_Md20_CrtStat_Val_write : Outport  Port=13
      settings: EnsureOutportIsVirtual=on
  IfVeSMSuStPassCmprtMd_Md21_CrtStat_Val_write : Outport  Port=14
      settings: EnsureOutportIsVirtual=on
  IfVeSMSuStPassCmprtMd_Md22_CrtStat_Val_write : Outport  Port=15
      settings: EnsureOutportIsVirtual=on
  IfVeSMSuStPassCmprtMd_Md23_CrtStat_Val_write : Outport  Port=16
      settings: EnsureOutportIsVirtual=on
  IfVeSMSuStPassCmprtMd_Md24_CrtStat_Val_write : Outport  Port=17
      settings: EnsureOutportIsVirtual=on
  IfVeSMSuStPassCmprtMd_Md25_CrtStat_Val_write : Outport  Port=18
      settings: EnsureOutportIsVirtual=on
  IfVeSMSuStPassCmprtMd_Md26_CrtStat_Val_write : Outport  Port=19
      settings: EnsureOutportIsVirtual=on
  IfVeSMSuStPassCmprtMd_Md27_CrtStat_Val_write : Outport  Port=20
      settings: EnsureOutportIsVirtual=on
  IfVeSMSuStPassCmprtMd_Md28_CrtStat_Val_write : Outport  Port=21
      settings: EnsureOutportIsVirtual=on
  IfVeSMSuStPassCmprtMd_Md29_CrtStat_Val_write : Outport  Port=22
      settings: EnsureOutportIsVirtual=on
  IfVeSMSuStPassCmprtMd_Md3_CrtStat_Val_write : Outport  Port=23
      settings: EnsureOutportIsVirtual=on
  IfVeSMSuStPassCmprtMd_Md30_CrtStat_Val_write : Outport  Port=24
      settings: EnsureOutportIsVirtual=on
  IfVeSMSuStPassCmprtMd_Md31_CrtStat_Val_write : Outport  Port=25
      settings: EnsureOutportIsVirtual=on
  IfVeSMSuStPassCmprtMd_Md32_CrtStat_Val_write : Outport  Port=26
      settings: EnsureOutportIsVirtual=on
  IfVeSMSuStPassCmprtMd_Md4_CrtStat_Val_write : Outport  Port=27
      settings: EnsureOutportIsVirtual=on
  IfVeSMSuStPassCmprtMd_Md5_CrtStat_Val_write : Outport  Port=28
      settings: EnsureOutportIsVirtual=on
  IfVeSMSuStPassCmprtMd_Md6_CrtStat_Val_write : Outport  Port=29
      settings: EnsureOutportIsVirtual=on
  IfVeSMSuStPassCmprtMd_Md7_CrtStat_Val_write : Outport  Port=30
      settings: EnsureOutportIsVirtual=on
  IfVeSMSuStPassCmprtMd_Md8_CrtStat_Val_write : Outport  Port=31
      settings: EnsureOutportIsVirtual=on
  IfVeSMSuStPassCmprtMd_Md9_CrtStat_Val_write : Outport  Port=32
      settings: EnsureOutportIsVirtual=on
  wires:
  MdXX_Stat_Md12_Stat_read/1 -> Data Type Conversion28/1
  MdXX_Stat_Md4_Stat_read/1 -> Data Type Conversion5/1
  MdXX_Stat_Md15_Stat_read/1 -> Data Type Conversion25/1
  MdXX_Stat_Md1_Stat_read/1 -> Data Type Conversion31/1
  MdXX_Stat_Md30_Stat_read/1 -> Data Type Conversion8/1
  MdXX_Stat_Md25_Stat_read/1 -> Data Type Conversion14/1
  MdXX_Stat_Md23_Stat_read/1 -> Data Type Conversion16/1
  MdXX_Stat_Md3_Stat_read/1 -> Data Type Conversion9/1
  MdXX_Stat_Md18_Stat_read/1 -> Data Type Conversion22/1
  MdXX_Stat_Md26_Stat_read/1 -> Data Type Conversion13/1
  MdXX_Stat_Md27_Stat_read/1 -> Data Type Conversion12/1
  MdXX_Stat_Md5_Stat_read/1 -> Data Type Conversion4/1
  MdXX_Stat_Md8_Stat_read/1 -> Data Type Conversion1/1
  MdXX_Stat_Md13_Stat_read/1 -> Data Type Conversion27/1
  MdXX_Stat_Md14_Stat_read/1 -> Data Type Conversion26/1
  MdXX_Stat_Md16_Stat_read/1 -> Data Type Conversion24/1
  MdXX_Stat_Md32_Stat_read/1 -> Data Type Conversion6/1
  MdXX_Stat_Md11_Stat_read/1 -> Data Type Conversion29/1
  MdXX_Stat_Md17_Stat_read/1 -> Data Type Conversion23/1
  MdXX_Stat_Md20_Stat_read/1 -> Data Type Conversion19/1
  MdXX_Stat_Md22_Stat_read/1 -> Data Type Conversion17/1
  MdXX_Stat_Md10_Stat_read/1 -> Data Type Conversion30/1
  MdXX_Stat_Md28_Stat_read/1 -> Data Type Conversion11/1
  MdXX_Stat_Md29_Stat_read/1 -> Data Type Conversion10/1
  MdXX_Stat_Md21_Stat_read/1 -> Data Type Conversion18/1
  MdXX_Stat_Md7_Stat_read/1 -> Data Type Conversion2/1
  MdXX_Stat_Md31_Stat_read/1 -> Data Type Conversion7/1
  MdXX_Stat_Md2_Stat_read/1 -> Data Type Conversion20/1
  MdXX_Stat_Md24_Stat_read/1 -> Data Type Conversion15/1
  MdXX_Stat_Md19_Stat_read/1 -> Data Type Conversion21/1
  MdXX_Stat_Md6_Stat_read/1 -> Data Type Conversion3/1
  MdXX_Stat_Md9_Stat_read/1 -> Data Type Conversion/1
  Data Type Conversion/1 -> IfVeSMSuStPassCmprtMd_Md9_CrtStat_Val_write/1
  Data Type Conversion1/1 -> IfVeSMSuStPassCmprtMd_Md8_CrtStat_Val_write/1
  Data Type Conversion2/1 -> IfVeSMSuStPassCmprtMd_Md7_CrtStat_Val_write/1
  Data Type Conversion3/1 -> IfVeSMSuStPassCmprtMd_Md6_CrtStat_Val_write/1
  Data Type Conversion4/1 -> IfVeSMSuStPassCmprtMd_Md5_CrtStat_Val_write/1
  Data Type Conversion5/1 -> IfVeSMSuStPassCmprtMd_Md4_CrtStat_Val_write/1
  Data Type Conversion6/1 -> IfVeSMSuStPassCmprtMd_Md32_CrtStat_Val_write/1
  Data Type Conversion7/1 -> IfVeSMSuStPassCmprtMd_Md31_CrtStat_Val_write/1
  Data Type Conversion8/1 -> IfVeSMSuStPassCmprtMd_Md30_CrtStat_Val_write/1
  Data Type Conversion9/1 -> IfVeSMSuStPassCmprtMd_Md3_CrtStat_Val_write/1
  Data Type Conversion10/1 -> IfVeSMSuStPassCmprtMd_Md29_CrtStat_Val_write/1
  Data Type Conversion11/1 -> IfVeSMSuStPassCmprtMd_Md28_CrtStat_Val_write/1
  Data Type Conversion12/1 -> IfVeSMSuStPassCmprtMd_Md27_CrtStat_Val_write/1
  Data Type Conversion13/1 -> IfVeSMSuStPassCmprtMd_Md26_CrtStat_Val_write/1
  Data Type Conversion14/1 -> IfVeSMSuStPassCmprtMd_Md25_CrtStat_Val_write/1
  Data Type Conversion15/1 -> IfVeSMSuStPassCmprtMd_Md24_CrtStat_Val_write/1
  Data Type Conversion16/1 -> IfVeSMSuStPassCmprtMd_Md23_CrtStat_Val_write/1
  Data Type Conversion17/1 -> IfVeSMSuStPassCmprtMd_Md22_CrtStat_Val_write/1
  Data Type Conversion18/1 -> IfVeSMSuStPassCmprtMd_Md21_CrtStat_Val_write/1
  Data Type Conversion19/1 -> IfVeSMSuStPassCmprtMd_Md20_CrtStat_Val_write/1
  Data Type Conversion20/1 -> IfVeSMSuStPassCmprtMd_Md2_CrtStat_Val_write/1
  Data Type Conversion21/1 -> IfVeSMSuStPassCmprtMd_Md19_CrtStat_Val_write/1
  Data Type Conversion22/1 -> IfVeSMSuStPassCmprtMd_Md18_CrtStat_Val_write/1
  Data Type Conversion23/1 -> IfVeSMSuStPassCmprtMd_Md17_CrtStat_Val_write/1
  Data Type Conversion24/1 -> IfVeSMSuStPassCmprtMd_Md16_CrtStat_Val_write/1
  Data Type Conversion25/1 -> IfVeSMSuStPassCmprtMd_Md15_CrtStat_Val_write/1
  Data Type Conversion26/1 -> IfVeSMSuStPassCmprtMd_Md14_CrtStat_Val_write/1
  Data Type Conversion27/1 -> IfVeSMSuStPassCmprtMd_Md13_CrtStat_Val_write/1
  Data Type Conversion28/1 -> IfVeSMSuStPassCmprtMd_Md12_CrtStat_Val_write/1
  Data Type Conversion29/1 -> IfVeSMSuStPassCmprtMd_Md11_CrtStat_Val_write/1
  Data Type Conversion30/1 -> IfVeSMSuStPassCmprtMd_Md10_CrtStat_Val_write/1
  Data Type Conversion31/1 -> IfVeSMSuStPassCmprtMd_Md1_CrtStat_Val_write/1
